simulink model "facedetection_raspi"  (R2021b)
settings: Solver=FixedStepAuto  StartTime=0.0  StopTime=10.0  RelTol=1e-3  EnableMultiTasking=on
libraries: raspberrypiBasiclib x4, raspberrypiNetworklib x3
settings Model: Creator=86139  LastModifiedBy=86139
settings SolverCC: PositivePriorityOrder=on
settings OptimizationCC: EnhancedBackFolding=on  PassReuseOutputArgsAs=Individual arguments  ZeroExternalMemoryAtStartup=off  ZeroInternalMemoryAtStartup=off  MaxStackSize=64  OptimizeBlockOrder=speed  DifferentSizesBufferReuse=on  OptimizationCustomize=off  EfficientTunableParamExpr=on
settings DebuggingCC: ParameterTunabilityLossMsg=error
settings HardwareCC: ProdBitPerPointer=32  ProdBitPerSizeT=32  ProdBitPerPtrDiffT=32  ProdLargestAtomicInteger=Long  ProdLargestAtomicFloat=Double  ProdWordSize=32  ProdLongLongMode=on  ProdHWDeviceType=ARM Compatible->ARM Cortex  UseEmbeddedCoderFeatures=off
settings RTWCC: Description=Embedded Coder  SystemTargetFile=ert.tlc  HardwareBoard=Raspberry Pi  TLCOptions="-aInlineSetEventsForThisBaseRateFcn=TLC_FALSE -aSuppressMultiTaskScheduler=TLC_FALSE  -aRateBasedStepFcn=0"  TemplateMakefile=ert_default_tmf  Toolchain=GNU GCC Embedded Linux  BuildConfiguration=Faster Runs
settings CodeAppCC: ForceParamTrailComments=on  IgnoreCustomStorageClasses=off  OperatorAnnotations=on  SimulinkDataObjDesc=on  SFDataObjDesc=on  InsertBlockDesc=on
settings ERTTargetCC: SupportNonInlinedSFcns=on  SupportVariableSizeSignals=on  ExtModeTransport=2  ExtModeStaticAlloc=on  ExtModeMexFile=ext_xcp  ExtModeIntrfLevel=Level2 - Open

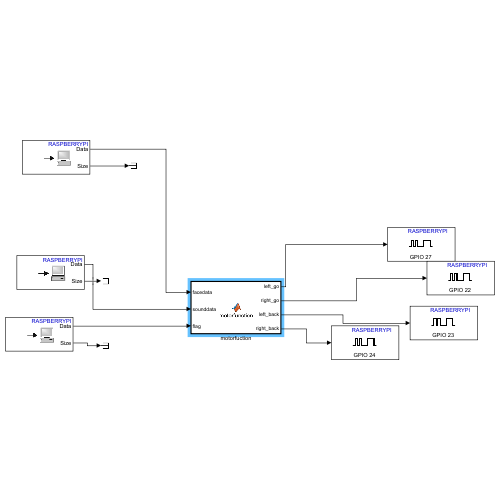
[thumbnail: Simulink's stored preview of the top-level diagram]
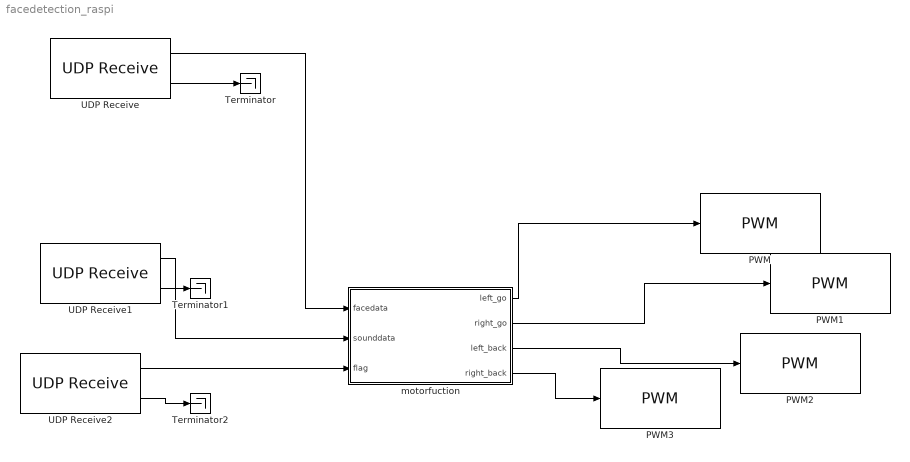
== system facedetection_raspi ==
  PWM : raspberrypiBasiclib/PWM  board=Pi 3 Model B  Pin_=27  Frequency=500  blockPlatform=Raspberry Pi
      settings: SourceProductBaseCode=RASPPI
  PWM1 : raspberrypiBasiclib/PWM  board=Pi 3 Model B  Pin_=22  Frequency=500  blockPlatform=Raspberry Pi
      settings: SourceProductBaseCode=RASPPI
  PWM2 : raspberrypiBasiclib/PWM  board=Pi 3 Model B  Pin_=23  Frequency=500  blockPlatform=Raspberry Pi
      settings: SourceProductBaseCode=RASPPI
  PWM3 : raspberrypiBasiclib/PWM  board=Pi 3 Model B  Pin_=24  Frequency=500  blockPlatform=Raspberry Pi
      settings: SourceProductBaseCode=RASPPI
  Terminator : Terminator
  Terminator1 : Terminator
  Terminator2 : Terminator
  UDP Receive : raspberrypiNetworklib/UDP Receive  localURL='0.0.0.0'  localPort=25000  remoteURL='0.0.0.0'  remotePort=-1  recvBufferSize=8192  signalDatatype=int8  dims=1  isVarSize=off  showBlockingTime=off  blockingTime=0  sampletime=0.01  blockPlatform=Raspberry Pi
      settings: SourceProductBaseCode=RASPPI
  UDP Receive1 : raspberrypiNetworklib/UDP Receive  localURL='0.0.0.0'  localPort=25001  remoteURL='0.0.0.0'  remotePort=-1  recvBufferSize=8192  signalDatatype=int8  dims=1  isVarSize=off  showBlockingTime=off  blockingTime=0  sampletime=0.01  blockPlatform=Raspberry Pi
      settings: SourceProductBaseCode=RASPPI
  UDP Receive2 : raspberrypiNetworklib/UDP Receive  localURL='0.0.0.0'  localPort=25002  remoteURL='0.0.0.0'  remotePort=-1  recvBufferSize=8192  signalDatatype=int8  dims=1  isVarSize=off  showBlockingTime=off  blockingTime=0  sampletime=0.01  blockPlatform=Raspberry Pi
      settings: SourceProductBaseCode=RASPPI
  motorfuction : MATLAB Function  TreatAsAtomicUnit=on
  wires:
  UDP Receive/2 -> Terminator/1
  UDP Receive/1 -> motorfuction/1(facedata)
  motorfuction/1(left_go) -> PWM/1
  motorfuction/2(right_go) -> PWM1/1
  motorfuction/3(left_back) -> PWM2/1
  motorfuction/4(right_back) -> PWM3/1
  UDP Receive1/1 -> motorfuction/2(sounddata)
  UDP Receive1/2 -> Terminator1/1
  UDP Receive2/1 -> motorfuction/3(flag)
  UDP Receive2/2 -> Terminator2/1

== matlab function facedetection_raspi/motorfuction ==
  data: facedata input; left_go output; right_go output; left_back output; right_back output; sounddata input; flag input
function [left_go,right_go,left_back,right_back] = motorfunction(facedata,sounddata,flag)

left_go = 0;
left_back = 0;
right_go = 0;
right_back = 0;


%sound 0-stop 1-go 2-left 3-right 4-back 5-others
%face 0-stop 1-go 2-left 3-right
if sounddata == 0
    if facedata == 0
        left_go = 0;
        right_go = 0;
        left_back = 0;
        right_back = 0;
    end
    if facedata == 1
        left_go = 0.4;
        right_go = 0.4;
        left_back = 0;
        right_back = 0;
    end
    if facedata == 2
        left_go = 0.2;
        right_go = 0.8;
        left_back = 0;
        right_back = 0;
    end
    if facedata == 3
        left_go = 0.8;
        right_go = 0.2;
        left_back = 0;
        right_back = 0;
    end
end
if sounddata == 1
    left_go = 1;
    right_go = 0.93;
    left_back = 0;
    right_back = 0;
end
if sounddata == 2
    left_go = 0.2;
    right_go = 1;
    left_back = 0;
    right_back = 0;
end
if sounddata == 3
    left_go = 1;
    right_go = 0.2;
    left_back = 0;
    right_back = 0;
end
if sounddata == 4
    left_go = 0;
    right_go = 0;
    left_back = 0.4;
    right_back = 0.4;
end
